simulink model "TorqueVectoringVehicleController"  (R2026b)
settings: Solver=FixedStepDiscrete  StopTime=1.0  FixedStep=TorqueVectoringControlSampleTime
undefined symbols (not defined in the file): TorqueVectoringBatterySOCUpperLimit, TorqueVectoringMaximumAcceleration, TorqueVectoringMaximumDeceleration, TorqueVectoringVehicleMass
settings Model: DataDictionary=VehicleData.sldd  Creator=Xu Dingyi  LastModifiedBy=29358
settings DebuggingCC: AlgebraicLoopMsg=error

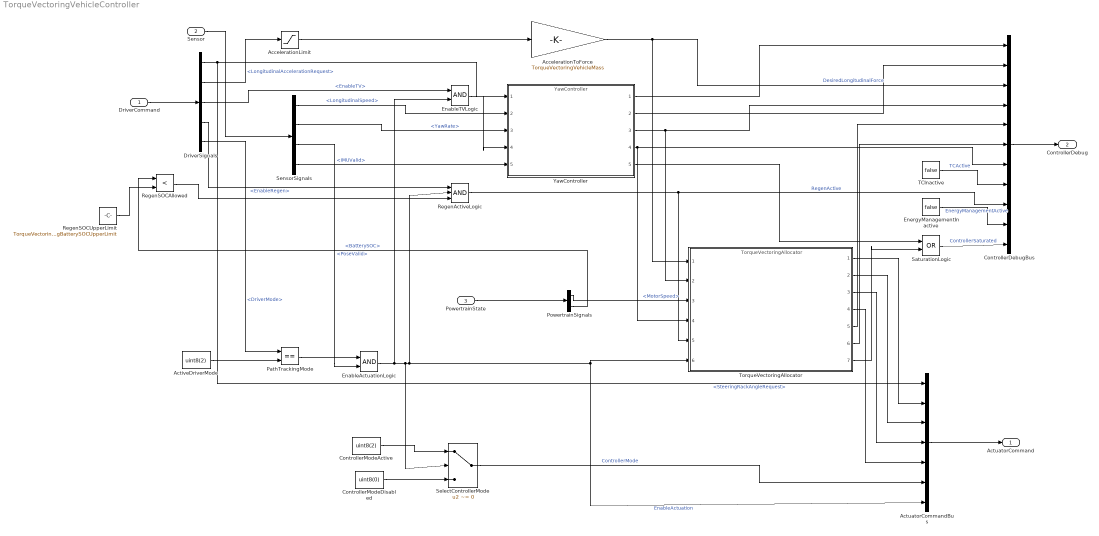
== system TorqueVectoringVehicleController ==
  DriverCommand : Inport  OutDataTypeStr=Bus: DriverCommandBus
  Sensor : Inport  Port=2  OutDataTypeStr=Bus: SensorBus
  PowertrainState : Inport  Port=3  OutDataTypeStr=Bus: PowertrainStateBus
  AccelerationLimit : Saturate  UpperLimit=TorqueVectoringMaximumAcceleration  LowerLimit=-TorqueVectoringMaximumDeceleration
  AccelerationToForce : Gain  Gain=TorqueVectoringVehicleMass
  ActiveDriverMode : Constant  Value=uint8(2)  OutDataTypeStr=uint8
  ActuatorCommandBus : BusCreator  Inputs=7  OutDataTypeStr=Bus: ActuatorCommandBus
  ControllerDebugBus : BusCreator  Inputs=11  OutDataTypeStr=Bus: ControllerDebugBus
  ControllerModeActive : Constant  Value=uint8(2)  OutDataTypeStr=uint8
  ControllerModeDisabled : Constant  Value=uint8(0)  OutDataTypeStr=uint8
  DriverSignals : BusSelector  OutputSignals=SteeringRackAngleRequest,LongitudinalAccelerationRequest,EnableTV,EnableRegen,DriverMode
  EnableActuationLogic : Logic  IconShape=distinctive  AllPortsSameDT=off  OutDataTypeStr=boolean
  EnableTVLogic : Logic  IconShape=distinctive  AllPortsSameDT=off  OutDataTypeStr=boolean
  EnergyManagementInactive : Constant  Value=false  OutDataTypeStr=boolean
  PathTrackingMode : RelationalOperator  Operator===
  PowertrainSignals : BusSelector  OutputSignals=MotorSpeed,BatterySOC
  RegenActiveLogic : Logic  Inputs=3  IconShape=distinctive  AllPortsSameDT=off  OutDataTypeStr=boolean
  RegenSOCAllowed : RelationalOperator  Operator=<
  RegenSOCUpperLimit : Constant  Value=TorqueVectoringBatterySOCUpperLimit
  SaturationLogic : Logic  Operator=OR  IconShape=distinctive  AllPortsSameDT=off  OutDataTypeStr=boolean
  SelectControllerMode : Switch  Criteria=u2 ~= 0
  SensorSignals : BusSelector  OutputSignals=LongitudinalSpeed,YawRate,PoseValid,IMUValid
  TCInactive : Constant  Value=false  OutDataTypeStr=boolean
  TorqueVectoringAllocator : ModelReference  ModelNameDialog=TorqueVectoringAllocator  ModelReferenceVersion=2.0
  YawController : ModelReference  ModelNameDialog=YawController  ModelReferenceVersion=1.4
  ActuatorCommand : Outport  OutDataTypeStr=Bus: ActuatorCommandBus
  ControllerDebug : Outport  Port=2  OutDataTypeStr=Bus: ControllerDebugBus
  wires:
  YawController/1 -> ControllerDebugBus/1
  Sensor/1 -> SensorSignals/1
  DriverSignals/4 -> RegenActiveLogic/1  "<EnableRegen>"
  SensorSignals/3 -> EnableActuationLogic/2  "<PoseValid>"
  DriverCommand/1 -> DriverSignals/1
  DriverSignals/2 -> AccelerationLimit/1  "<LongitudinalAccelerationRequest>"
  DriverSignals/5 -> PathTrackingMode/1  "<DriverMode>"
  EnergyManagementInactive/1 -> ControllerDebugBus/10  "EnergyManagementActive"
  DriverSignals/3 -> EnableTVLogic/1  "<EnableTV>"
  YawController/5 -> SaturationLogic/1
  SensorSignals/2 -> YawController/3  "<YawRate>"
  DriverSignals/1 -> ActuatorCommandBus/1, YawController/1  "<SteeringRackAngleRequest>"
  ActiveDriverMode/1 -> PathTrackingMode/2
  TorqueVectoringAllocator/3 -> ActuatorCommandBus/4
  AccelerationLimit/1 -> AccelerationToForce/1
  TorqueVectoringAllocator/5 -> ControllerDebugBus/5
  SensorSignals/1 -> YawController/2  "<LongitudinalSpeed>"
  SensorSignals/4 -> YawController/5  "<IMUValid>"
  PathTrackingMode/1 -> EnableActuationLogic/1
  EnableActuationLogic/1 -> TorqueVectoringAllocator/6, ActuatorCommandBus/7, RegenActiveLogic/2, SelectControllerMode/2, EnableTVLogic/2  "EnableActuation"
  ControllerModeActive/1 -> SelectControllerMode/1
  PowertrainSignals/1 -> TorqueVectoringAllocator/3  "<MotorSpeed>"
  PowertrainState/1 -> PowertrainSignals/1
  ControllerModeDisabled/1 -> SelectControllerMode/3
  EnableTVLogic/1 -> YawController/4
  RegenActiveLogic/1 -> ControllerDebugBus/9, TorqueVectoringAllocator/5  "RegenActive"
  SelectControllerMode/1 -> ActuatorCommandBus/6  "ControllerMode"
  AccelerationToForce/1 -> TorqueVectoringAllocator/1, ControllerDebugBus/3  "DesiredLongitudinalForce"
  YawController/2 -> ControllerDebugBus/2
  YawController/3 -> ControllerDebugBus/4, TorqueVectoringAllocator/2
  YawController/4 -> ControllerDebugBus/7, TorqueVectoringAllocator/4
  TorqueVectoringAllocator/1 -> ActuatorCommandBus/2
  TorqueVectoringAllocator/2 -> ActuatorCommandBus/3
  TorqueVectoringAllocator/4 -> ActuatorCommandBus/5
  TorqueVectoringAllocator/6 -> ControllerDebugBus/6
  TorqueVectoringAllocator/7 -> SaturationLogic/2
  TCInactive/1 -> ControllerDebugBus/8  "TCActive"
  SaturationLogic/1 -> ControllerDebugBus/11  "ControllerSaturated"
  ActuatorCommandBus/1 -> ActuatorCommand/1
  ControllerDebugBus/1 -> ControllerDebug/1
  RegenSOCUpperLimit/1 -> RegenSOCAllowed/2
  PowertrainSignals/2 -> RegenSOCAllowed/1  "<BatterySOC>"
  RegenSOCAllowed/1 -> RegenActiveLogic/3
